simulink model "system"  (Simulink 7.0)
settings: Solver=ode45  StartTime=0.0  StopTime=10.0  RelTol=1e-3
settings Model: Creator=12345678  LastModifiedBy=12345678

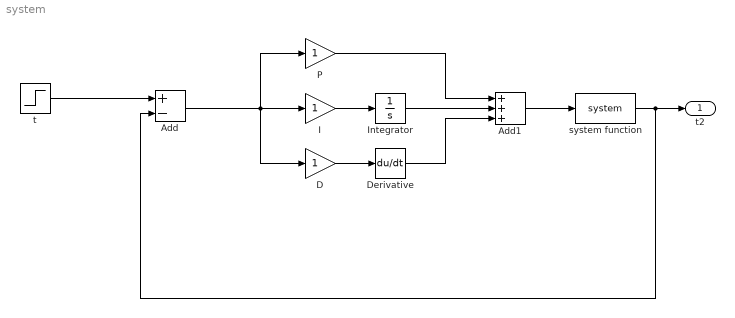
== system system ==
  Add : Sum  Inputs=+-  OutDataType=sfix(16)  OutScaling=2^-10
  Add1 : Sum  Inputs=+++  OutDataType=sfix(16)  OutScaling=2^-10
  D : Gain  ParameterDataType=sfix(16)  ParameterScaling=2^0  OutDataType=sfix(16)  OutScaling=2^0
  Derivative : Derivative
  I : Gain  ParameterDataType=sfix(16)  ParameterScaling=2^0  OutDataType=sfix(16)  OutScaling=2^0
  Integrator : Integrator
  P : Gain  ParameterDataType=sfix(16)  ParameterScaling=2^0  OutDataType=sfix(16)  OutScaling=2^0
  system function : S-Function
  t : Step  SampleTime=0
  t2 : Outport  OutDataType=sfix(16)  OutScaling=2^0
  wires:
  Add/1 -> I/1, P/1, D/1
  t/1 -> Add/1
  D/1 -> Derivative/1
  I/1 -> Integrator/1
  Derivative/1 -> Add1/3
  Integrator/1 -> Add1/2
  P/1 -> Add1/1
  Add1/1 -> system function/1
  system function/1 -> t2/1, Add/2
